simulink model "Project3_System_partB_R2017a"  (R2017a)
settings: Solver=VariableStepAuto  StartTime=0.0  StopTime=10  FixedStep=.001  MaxStep=.001  RelTol=1e-6  EnableMultiTasking=on
values from neighbouring files (symbols this model uses):
  Kd = 700    [SimRun.m]
  Kp = 1000    [SimRun.m]
  n = link.inertia*(iwdot) + cross(iw, link.inertia*iw)    [newtonEuler.m]
  points = points3D    [SimRun.m]
  th_last = [0;-pi/2;0;0;0;0]    [SimRun.m]    (also in fcn.m)
  transPercent = 0.025    [SimRun.m]
(part 4 of 4)

== matlab function Project3_System_partB_R2017a/MATLAB Function ==
  data: theta input; theta_ddot input; torque output; theta_dot input
function torque = newton_euler( theta, theta_ddot, theta_dot )
%#codegen
coder.extrinsic('evalin');
coder.extrinsic('newtonEuler');

persistent linkList boundry_conditions;

if isempty(linkList)
    linkList = evalin('base','linkList');
    boundry_conditions.base_angular_velocity = [0;0;0];
    boundry_conditions.base_angular_acceleration = [0;0;0];
    boundry_conditions.base_linear_acceleration = [0;0;9.8];
    boundry_conditions.distal_force = [0;0;0];
    boundry_conditions.distal_torque = [0;0;0];
end

% theta(2) = theta(2)-pi/2; % put in DH frame
torque = zeros(6,1);
torque = newtonEuler(linkList,theta,theta_dot,theta_ddot,boundry_conditions);


end

== matlab function Project3_System_partB_R2017a/ABB Arm Dynamics/Laser Tracking ==
  data: theta input; pose output
function pose = laserTracker(theta)
%#codegen
coder.extrinsic('evalin');
persistent Sim_Exact;

if isempty(Sim_Exact)
    Sim_Exact = evalin('base','Sim_Exact');
end


th1 = theta(1);
th2 = theta(2);
th3 = theta(3);
th4 = theta(4);
th5 = theta(5);
th6 = theta(6);


if(Sim_Exact)
    pose = [ sin(th6)*(cos(th4)*sin(th1) + sin(th4)*(cos(th1)*sin(th2)*sin(th3) - cos(th1)*cos(th2)*cos(th3))) + cos(th6)*(cos(th5)*(sin(th1)*sin(th4) - cos(th4)*(cos(th1)*sin(th2)*sin(th3) - cos(th1)*cos(th2)*cos(th3))) - sin(th5)*(cos(th1)*cos(th2)*sin(th3) + cos(th1)*cos(th3)*sin(th2))), cos(th6)*(cos(th4)*sin(th1) + sin(th4)*(cos(th1)*sin(th2)*sin(th3) - cos(th1)*cos(th2)*cos(th3))) - sin(th6)*(cos(th5)*(sin(th1)*sin(th4) - cos(th4)*(cos(th1)*sin(th2)*sin(th3) - cos(th1)*cos(th2)*cos(th3))) - sin(th5)*(cos(th1)*cos(th2)*sin(th3) + cos(th1)*cos(th3)*sin(th2))), - sin(th5)*(sin(th1)*sin(th4) - cos(th4)*(cos(th1)*sin(th2)*sin(th3) - cos(th1)*cos(th2)*cos(th3))) - cos(th5)*(cos(th1)*cos(th2)*sin(th3) + cos(th1)*cos(th3)*sin(th2)), (27*cos(th1)*cos(th2))/100 - (9*sin(th5)*(sin(th1)*sin(th4) - cos(th4)*(cos(th1)*sin(th2)*sin(th3) - cos(th1)*cos(th2)*cos(th3))))/125 - (9*cos(th5)*(cos(th1)*cos(th2)*sin(th3) + cos(th1)*cos(th3)*sin(th2)))/125 - (7*cos(th1)*sin(th2)*sin(th3))/100 + (7*cos(th1)*cos(th2)*cos(th3))/100 - (151*cos(th1)*cos(th2)*sin(th3))/500 - (151*cos(th1)*cos(th3)*sin(th2))/500;
        - sin(th6)*(cos(th1)*cos(th4) - sin(th4)*(sin(th1)*sin(th2)*sin(th3) - cos(th2)*cos(th3)*sin(th1))) - cos(th6)*(cos(th5)*(cos(th1)*sin(th4) + cos(th4)*(sin(th1)*sin(th2)*sin(th3) - cos(th2)*cos(th3)*sin(th1))) + sin(th5)*(cos(th2)*sin(th1)*sin(th3) + cos(th3)*sin(th1)*sin(th2))), sin(th6)*(cos(th5)*(cos(th1)*sin(th4) + cos(th4)*(sin(th1)*sin(th2)*sin(th3) - cos(th2)*cos(th3)*sin(th1))) + sin(th5)*(cos(th2)*sin(th1)*sin(th3) + cos(th3)*sin(th1)*sin(th2))) - cos(th6)*(cos(th1)*cos(th4) - sin(th4)*(sin(th1)*sin(th2)*sin(th3) - cos(th2)*cos(th3)*sin(th1))), sin(th5)*(cos(th1)*sin(th4) + cos(th4)*(sin(th1)*sin(th2)*sin(th3) - cos(th2)*cos(th3)*sin(th1))) - cos(th5)*(cos(th2)*sin(th1)*sin(th3) + cos(th3)*sin(th1)*sin(th2)), (27*cos(th2)*sin(th1))/100 + (9*sin(th5)*(cos(th1)*sin(th4) + cos(th4)*(sin(th1)*sin(th2)*sin(th3) - cos(th2)*cos(th3)*sin(th1))))/125 - (9*cos(th5)*(cos(th2)*sin(th1)*sin(th3) + cos(th3)*sin(th1)*sin(th2)))/125 - (151*cos(th2)*sin(th1)*sin(th3))/500 - (151*cos(th3)*sin(th1)*sin(th2))/500 - (7*sin(th1)*sin(th2)*sin(th3))/100 + (7*cos(th2)*cos(th3)*sin(th1))/100;
        sin(th4)*sin(th6)*(cos(th2)*sin(th3) + cos(th3)*sin(th2)) - cos(th6)*(sin(th5)*(cos(th2)*cos(th3) - sin(th2)*sin(th3)) + cos(th4)*cos(th5)*(cos(th2)*sin(th3) + cos(th3)*sin(th2))), sin(th6)*(sin(th5)*(cos(th2)*cos(th3) - sin(th2)*sin(th3)) + cos(th4)*cos(th5)*(cos(th2)*sin(th3) + cos(th3)*sin(th2))) + cos(th6)*sin(th4)*(cos(th2)*sin(th3) + cos(th3)*sin(th2)), cos(th4)*sin(th5)*(cos(th2)*sin(th3) + cos(th3)*sin(th2)) - cos(th5)*(cos(th2)*cos(th3) - sin(th2)*sin(th3)), (151*sin(th2)*sin(th3))/500 - (151*cos(th2)*cos(th3))/500 - (7*cos(th2)*sin(th3))/100 - (7*cos(th3)*sin(th2))/100 - (27*sin(th2))/100 - (9*cos(th5)*(cos(th2)*cos(th3) - sin(th2)*sin(th3)))/125 + (9*cos(th4)*sin(th5)*(cos(th2)*sin(th3) + cos(th3)*sin(th2)))/125 + 29/100;
        0, 0, 0, 1];
else
    
    pose = [ sin(th6)*(cos(th4)*sin(th1) + sin(th4)*(cos(th1)*sin(th2)*sin(th3) - cos(th1)*cos(th2)*cos(th3))) + cos(th6)*(cos(th5)*(sin(th1)*sin(th4) - cos(th4)*(cos(th1)*sin(th2)*sin(th3) - cos(th1)*cos(th2)*cos(th3))) - sin(th5)*(cos(th1)*cos(th2)*sin(th3) + cos(th1)*cos(th3)*sin(th2))), cos(th6)*(cos(th4)*sin(th1) + sin(th4)*(cos(th1)*sin(th2)*sin(th3) - cos(th1)*cos(th2)*cos(th3))) - sin(th6)*(cos(th5)*(sin(th1)*sin(th4) - cos(th4)*(cos(th1)*sin(th2)*sin(th3) - cos(th1)*cos(th2)*cos(th3))) - sin(th5)*(cos(th1)*cos(th2)*sin(th3) + cos(th1)*cos(th3)*sin(th2))), - sin(th5)*(sin(th1)*sin(th4) - cos(th4)*(cos(th1)*sin(th2)*sin(th3) - cos(th1)*cos(th2)*cos(th3))) - cos(th5)*(cos(th1)*cos(th2)*sin(th3) + cos(th1)*cos(th3)*sin(th2)), (151838081588107*cos(th1)*cos(th2))/562949953421312 - (123928564092639*sin(th1))/72057594037927936 - (7184037743251309*cos(th1))/36893488147419103232 - (7330531551818703*cos(th4)*sin(th1))/36893488147419103232 - (5489399374888815*sin(th1)*sin(th4))/9223372036854775808 + (970893499285375*cos(th5)*(sin(th1)*sin(th4) - cos(th4)*(cos(th1)*sin(th2)*sin(th3) - cos(th1)*cos(th2)*cos(th3))))/9223372036854775808 - (5192391675427195*sin(th5)*(sin(th1)*sin(th4) - cos(th4)*(cos(th1)*sin(th2)*sin(th3) - cos(th1)*cos(th2)*cos(th3))))/72057594037927936 + (1663072680156839*sin(th6)*(cos(th4)*sin(th1) + sin(th4)*(cos(th1)*sin(th2)*sin(th3) - cos(th1)*cos(th2)*cos(th3))))/2305843009213693952 + (1663072680156839*cos(th6)*(cos(th5)*(sin(th1)*sin(th4) - cos(th4)*(cos(th1)*sin(th2)*sin(th3) - cos(th1)*cos(th2)*cos(th3))) - sin(th5)*(cos(th1)*cos(th2)*sin(th3) + cos(th1)*cos(th3)*sin(th2))))/2305843009213693952 + (5489399374888815*cos(th4)*(cos(th1)*sin(th2)*sin(th3) - cos(th1)*cos(th2)*cos(th3)))/9223372036854775808 - (5192391675427195*cos(th5)*(cos(th1)*cos(th2)*sin(th3) + cos(th1)*cos(th3)*sin(th2)))/72057594037927936 - (7330531551818703*sin(th4)*(cos(th1)*sin(th2)*sin(th3) - cos(th1)*cos(th2)*cos(th3)))/36893488147419103232 - (970893499285375*sin(th5)*(cos(th1)*cos(th2)*sin(th3) + cos(th1)*cos(th3)*sin(th2)))/9223372036854775808 - (1259578569946919*cos(th1)*sin(th2)*sin(th3))/18014398509481984 + (1259578569946919*cos(th1)*cos(th2)*cos(th3))/18014398509481984 - (5430591396830085*cos(th1)*cos(th2)*sin(th3))/18014398509481984 - (5430591396830085*cos(th1)*cos(th3)*sin(th2))/18014398509481984;
        - sin(th6)*(cos(th1)*cos(th4) - sin(th4)*(sin(th1)*sin(th2)*sin(th3) - cos(th2)*cos(th3)*sin(th1))) - cos(th6)*(cos(th5)*(cos(th1)*sin(th4) + cos(th4)*(sin(th1)*sin(th2)*sin(th3) - cos(th2)*cos(th3)*sin(th1))) + sin(th5)*(cos(th2)*sin(th1)*sin(th3) + cos(th3)*sin(th1)*sin(th2))), sin(th6)*(cos(th5)*(cos(th1)*sin(th4) + cos(th4)*(sin(th1)*sin(th2)*sin(th3) - cos(th2)*cos(th3)*sin(th1))) + sin(th5)*(cos(th2)*sin(th1)*sin(th3) + cos(th3)*sin(th1)*sin(th2))) - cos(th6)*(cos(th1)*cos(th4) - sin(th4)*(sin(th1)*sin(th2)*sin(th3) - cos(th2)*cos(th3)*sin(th1))), sin(th5)*(cos(th1)*sin(th4) + cos(th4)*(sin(th1)*sin(th2)*sin(th3) - cos(th2)*cos(th3)*sin(th1))) - cos(th5)*(cos(th2)*sin(th1)*sin(th3) + cos(th3)*sin(th1)*sin(th2)), (123928564092639*cos(th1))/72057594037927936 - (7184037743251309*sin(th1))/36893488147419103232 + (7330531551818703*cos(th1)*cos(th4))/36893488147419103232 + (151838081588107*cos(th2)*sin(th1))/562949953421312 + (5489399374888815*cos(th1)*sin(th4))/9223372036854775808 - (970893499285375*cos(th5)*(cos(th1)*sin(th4) + cos(th4)*(sin(th1)*sin(th2)*sin(th3) - cos(th2)*cos(th3)*sin(th1))))/9223372036854775808 + (5192391675427195*sin(th5)*(cos(th1)*sin(th4) + cos(th4)*(sin(th1)*sin(th2)*sin(th3) - cos(th2)*cos(th3)*sin(th1))))/72057594037927936 - (1663072680156839*sin(th6)*(cos(th1)*cos(th4) - sin(th4)*(sin(th1)*sin(th2)*sin(th3) - cos(th2)*cos(th3)*sin(th1))))/2305843009213693952 + (5489399374888815*cos(th4)*(sin(th1)*sin(th2)*sin(th3) - cos(th2)*cos(th3)*sin(th1)))/9223372036854775808 - (5192391675427195*cos(th5)*(cos(th2)*sin(th1)*sin(th3) + cos(th3)*sin(th1)*sin(th2)))/72057594037927936 - (1663072680156839*cos(th6)*(cos(th5)*(cos(th1)*sin(th4) + cos(th4)*(sin(th1)*sin(th2)*sin(th3) - cos(th2)*cos(th3)*sin(th1))) + sin(th5)*(cos(th2)*sin(th1)*sin(th3) + cos(th3)*sin(th1)*sin(th2))))/2305843009213693952 - (7330531551818703*sin(th4)*(sin(th1)*sin(th2)*sin(th3) - cos(th2)*cos(th3)*sin(th1)))/36893488147419103232 - (970893499285375*sin(th5)*(cos(th2)*sin(th1)*sin(th3) + cos(th3)*sin(th1)*sin(th2)))/9223372036854775808 - (5430591396830085*cos(th2)*sin(th1)*sin(th3))/18014398509481984 - (5430591396830085*cos(th3)*sin(th1)*sin(th2))/18014398509481984 - (1259578569946919*sin(th1)*sin(th2)*sin(th3))/18014398509481984 + (1259578569946919*cos(th2)*cos(th3)*sin(th1))/18014398509481984;
        sin(th4)*sin(th6)*(cos(th2)*sin(th3) + cos(th3)*sin(th2)) - cos(th6)*(sin(th5)*(cos(th2)*cos(th3) - sin(th2)*sin(th3)) + cos(th4)*cos(th5)*(cos(th2)*sin(th3) + cos(th3)*sin(th2))), sin(th6)*(sin(th5)*(cos(th2)*cos(th3) - sin(th2)*sin(th3)) + cos(th4)*cos(th5)*(cos(th2)*sin(th3) + cos(th3)*sin(th2))) + cos(th6)*sin(th4)*(cos(th2)*sin(th3) + cos(th3)*sin(th2)), cos(th4)*sin(th5)*(cos(th2)*sin(th3) + cos(th3)*sin(th2)) - cos(th5)*(cos(th2)*cos(th3) - sin(th2)*sin(th3)), (5430591396830085*sin(th2)*sin(th3))/18014398509481984 - (5430591396830085*cos(th2)*cos(th3))/18014398509481984 - (1259578569946919*cos(th2)*sin(th3))/18014398509481984 - (1259578569946919*cos(th3)*sin(th2))/18014398509481984 - (1663072680156839*cos(th6)*(sin(th5)*(cos(th2)*cos(th3) - sin(th2)*sin(th3)) + cos(th4)*cos(th5)*(cos(th2)*sin(th3) + cos(th3)*sin(th2))))/2305843009213693952 - (151838081588107*sin(th2))/562949953421312 + (5489399374888815*cos(th4)*(cos(th2)*sin(th3) + cos(th3)*sin(th2)))/9223372036854775808 - (5192391675427195*cos(th5)*(cos(th2)*cos(th3) - sin(th2)*sin(th3)))/72057594037927936 - (7330531551818703*sin(th4)*(cos(th2)*sin(th3) + cos(th3)*sin(th2)))/36893488147419103232 - (970893499285375*sin(th5)*(cos(th2)*cos(th3) - sin(th2)*sin(th3)))/9223372036854775808 - (970893499285375*cos(th4)*cos(th5)*(cos(th2)*sin(th3) + cos(th3)*sin(th2)))/9223372036854775808 + (5192391675427195*cos(th4)*sin(th5)*(cos(th2)*sin(th3) + cos(th3)*sin(th2)))/72057594037927936 + (1663072680156839*sin(th4)*sin(th6)*(cos(th2)*sin(th3) + cos(th3)*sin(th2)))/2305843009213693952 + 325695105792877/1125899906842624;
        0, 0, 0, 1];
end

== matlab function Project3_System_partB_R2017a/MATLAB Function1 ==
  data: t input; traj output; points input; n input
function traj = trajectory(t,points,n)
d1 = 0.29;
a2 = 0.270;
a3 = 0.070;
d4 = 0.302;
d6 = 0.072;

rcom1 = [0;-d1/2;0];
rcom2 = [-a2/2;0;0];
rcom3 = [-a3/2;0;0];
rcom4 = [0;-d4/2;0];
rcom5 = [0;0;0];
rcom6 = [0; -d6/2;0];

rad1 = .2/2; h1 = d1;   m1 = 8050*h1*rad1^2*pi;
rad2 = .15/2; h2 = a2;   m2 = 8050*h2*rad2^2*pi;
rad3 = .1/2; h3 = a3;  m3 = 8050*h3*rad3^2*pi;
rad4 = .1/2; h4 = d4;  m4 = 8050*h4*rad4^2*pi;
rad5 = .05/2; h5 = .125; m5 = 8050*h5*rad5^2*pi;
rad6 = .05/2; h6 = d6;  m6 = 8050*h6*rad6^2*pi;

J1 = diag(m1*[1/12*(3*rad1^2+h1^2),rad1^2/2,1/12*(3*rad1^2+h1^2)]);
J2 = diag(m2*[rad2^2/2,1/12*(3*rad2^2+h2^2),1/12*(3*rad2^2+h2^2)]);
J3 = diag(m3*[rad3^2/2,1/12*(3*rad3^2+h3^2),1/12*(3*rad3^2+h3^2)]);
J4 = diag(m4*[1/12*(3*rad4^2+h4^2),rad4^2/2,1/12*(3*rad4^2+h4^2)]);
J5 = diag(m5*[1/12*(3*rad5^2+h5^2),rad5^2/2,1/12*(3*rad5^2+h5^2)]);
J6 = diag(m6*[1/12*(3*rad6^2+h6^2),rad6^2/2,1/12*(3*rad6^2+h6^2)]);

L1 = createLink(0,d1,-pi/2,[],rcom1, m1,J1);
L2 = createLink(a2,0,0,[],rcom2, m2,J2);
L3 = createLink(a3,0,-pi/2,[],rcom3, m3,J3);
L4 = createLink(0,d4,pi/2,[],rcom4, m4,J4);
L5 = createLink(0,0,-pi/2,[],rcom5, m5,J5);
L6 = createLink(0,d6,0,[],rcom6, m6,J6);

linkList = [L1;L2;L3;L4;L5;L6]';

traj=zeros(length(t),8);
traj1=zeros(length(t),8);
% [p,~]=size(points);
% th=zeros(p+3,6);
% th(1,:)=[0;pi/2;0;0;0;0]';
z_vec=n;
Q=zeros(4,length(t));
Q1=zeros(4,length(t));
% H_ini=dhFwdKine(linkList,th(1,:));
% R_ini=H_ini(1:3,1:3);
Q1(:,1) = rot2Quat(eye(3));
Q(:,1)=Q1(:,1)/norm(Q1(:,1));
diff=(points(2,:)-points(1,:));
x_vec=diff'/norm(diff);
y_vec=cpMap(z_vec)*x_vec;
R=[x_vec y_vec z_vec];
traj1(1,:)=[t(1),[0 0 0],Q(:,1)'];
% [th1,th2,th3,th4,th5,th6 ,~]=abbInvKine([eye(3) points(1,:)'],-1*th(1,:)');
% th(2,:)=[th1,th2,th3,th4,th5,th6];
% th(3,:)=[th1,th2,th3,th4,th5,th6];
% H_i=dhFwdKine(linkList,th(2,:)');
% R_i=H_i(1:3,1:3);
Q1(:,2) = rot2Quat(R);
Q(:,2)=Q1(:,2)/norm(Q1(:,2));
traj1(2,:)=[t(2),points(1,:),Q(:,2)'];
traj1(3,:)=[t(3),points(1,:),Q(:,2)'];
for i=3:length(t)-2
    diff=points(i-1,:)-points(i-2,:);
    x_vec=diff'/norm(diff);
    y_vec=cpMap(z_vec)*x_vec;
    R=[x_vec y_vec z_vec];
% [th1,th2,th3,th4,th5,th6 ,~]=abbInvKine([eye(3) points(i-1,:)'],th(i,:)');
% th(i+1,:)=[th1,th2,th3,th4,th5,th6];
% H_i=dhFwdKine(linkList,th(i,:)');
% R_i=H_i(1:3,1:3);
Q1(:,i) = rot2Quat(R);
Q(:,i)=Q1(:,i)/norm(Q1(:,i));
if (Q(:,i-1)')*Q(:,i) < 0
    Q=-1*Q;
end
traj1(i+1,:)=[t(i+1),points(i-1,:),Q(:,i)'];
end
traj1(24,:)=[t(24),points(21,:),Q(:,i)'];
traj=traj1;
end

== matlab function Project3_System_partB_R2017a/MATLAB Function2 ==
  data: time input double; T_des output double; x_des_ddot output; traj input double; transPercent input double; x_des_dot output double
function [T_des,x_des_ddot,x_des_dot] = constAccelInterp(time,traj,transPercent)
t = traj(:,1);
[n,m] = size(traj);
x1 = zeros(1,7);
x1_dot = zeros(1,7);
x1_ddot = zeros(1,7);
omega=zeros(3,1);
omega1=zeros(3,1);
x_des=zeros(6,1);
x_dot_des=zeros(6,1);
q1=zeros(4,1);
q=zeros(4,1);

for j = 2:n-1
    if j-1==1 && time>=t(j-1,1) && time<=(t(j-1,1)+transPercent)
        for i = 2:m
            x1(1,i-1) = traj(j-1,i) + (((traj(j,i)-traj(j-1,i))*((time-t(j-1,1)+transPercent)^2))/(4*transPercent*(t(j,1)-t(j-1,1))));
            x1_dot(1,i-1) = (((traj(j,i)-traj(j-1,i))*(time-t(j-1,1)+transPercent))/(2*transPercent*(t(j,1)-t(j-1,1))));
            x1_ddot(1,i-1) = ((traj(j,i)-traj(j-1,i))/(2*transPercent*(t(j,1)-t(j-1,1))));
        end
        break;
    elseif j+1==n && time>=(t(j+1,1)-transPercent) && time<=t(j+1,1)
        for i = 2:m
            x1(1,i-1) = traj(j+1,i) - (((traj(j+1,i)-traj(j,i))*((time-t(j+1,1)-transPercent)^2))/(4*transPercent*(t(j+1,1)-t(j,1))));
            x1_dot(1,i-1) = -(((traj(j+1,i)-traj(j,i))*(time-t(j+1,1)-transPercent))/(2*transPercent*(t(j+1,1)-t(j,1))));
            x1_ddot(1,i-1) = -((traj(j+1,i)-traj(j,i))/(2*transPercent*(t(j+1,1)-t(j,1))));
        end
        break;
    elseif time>=(t(j-1,1)+transPercent) && time<=(t(j,1)-transPercent)
        for i = 2:m
            x1(1,i-1) = traj(j,i)-(((t(j,1)-time)*(traj(j,i)- traj(j-1,i)))/(t(j,1)-t(j-1,1)));
            x1_dot(1,i-1) = (traj(j,i)-traj(j-1,i))/(t(j,1)-t(j-1,1));
            x1_ddot(1,i-1) = 0.0;
        end
        break;
    elseif time>=(t(j,1)-transPercent) && time<=(t(j,1)+transPercent)
        for i = 2:m
            x1(1,i-1) = traj(j,i) - ...
                (((traj(j,i)-traj(j-1,i))*((time-t(j,1)-transPercent)^2))/(4*transPercent*(t(j,1)-t(j-1,1)))) + (((traj(j+1,i)-traj(j,i))*((time-t(j,1)+transPercent)^2))/(4*transPercent*(t(j+1,1)-t(j,1))));
            x1_dot(1,i-1) = -(((traj(j,i)-traj(j-1,i))*(time-t(j,1)-transPercent))/(2*transPercent*(t(j,1)-t(j-1,1)))) + (((traj(j+1,i)-traj(j,i))*(time-t(j,1)+transPercent))/(2*transPercent*(t(j+1,1)-t(j,1))));
            x1_ddot(1,i-1) = -((traj(j,i)-traj(j-1,i))/(2*transPercent*(t(j,1)-t(j-1,1)))) + ((traj(j+1,i)-traj(j,i))/(2*transPercent*(t(j+1,1)-t(j,1))));
        end
        break;
    elseif time>=(t(j,1)+transPercent) && time<=(t(j+1,1)-transPercent)
        for i = 2:m
            x1(1,i-1) = traj(j,i)+(((time-t(j,1))*(traj(j+1,i)-traj(j,i)))/(t(j+1,1)-t(j,1)));
            x1_dot(1,i-1) = (traj(j+1,i)-traj(j,i))/(t(j+1,1)-t(j,1));
            x1_ddot(1,i-1) = 0;
        end
        break;
        
    end
end
q1(:,1)=x1(4:7)';
R=quat2Rot(q1);
% [k,theta]=rot2AngleAxis(R);
% omega=k*theta;
T_des=[R x1(1:3)';0 0 0 1];
% x_des=[x1(1:3),omega']';
dq=x1_dot(4:7);
omega1=2*[dq(2:4)' (dq(1)*eye(3))+cpMap(dq(2:4))]*dq';
x_des_dot=[x1_dot(1:3)';omega1]';
dq1=x1_ddot(4:7);
omega_dot=2*[dq1(2:4)' (dq1(1)*eye(3))+cpMap(dq1(2:4))]*dq1';
x_des_ddot=[x1_ddot(1:3)';omega_dot]';
end

== matlab function Project3_System_partB_R2017a/MATLAB Function3 ==
  data: Jv output; paramList input; paramRateList input; Jv_inv output; JvDot output
function [Jv,Jv_inv,JvDot] = Jacobian(paramList,paramRateList)

d1 = 0.29;
a2 = 0.270;
a3 = 0.070;
d4 = 0.302;
d6 = 0.072;

rcom1 = [0;-d1/2;0];
rcom2 = [-a2/2;0;0];
rcom3 = [-a3/2;0;0];
rcom4 = [0;-d4/2;0];
rcom5 = [0;0;0];
rcom6 = [0; -d6/2;0];

rad1 = .2/2; h1 = d1;   m1 = 8050*h1*rad1^2*pi;
rad2 = .15/2; h2 = a2;   m2 = 8050*h2*rad2^2*pi;
rad3 = .1/2; h3 = a3;  m3 = 8050*h3*rad3^2*pi;
rad4 = .1/2; h4 = d4;  m4 = 8050*h4*rad4^2*pi;
rad5 = .05/2; h5 = .125; m5 = 8050*h5*rad5^2*pi;
rad6 = .05/2; h6 = d6;  m6 = 8050*h6*rad6^2*pi;

J1 = diag(m1*[1/12*(3*rad1^2+h1^2),rad1^2/2,1/12*(3*rad1^2+h1^2)]);
J2 = diag(m2*[rad2^2/2,1/12*(3*rad2^2+h2^2),1/12*(3*rad2^2+h2^2)]);
J3 = diag(m3*[rad3^2/2,1/12*(3*rad3^2+h3^2),1/12*(3*rad3^2+h3^2)]);
J4 = diag(m4*[1/12*(3*rad4^2+h4^2),rad4^2/2,1/12*(3*rad4^2+h4^2)]);
J5 = diag(m5*[1/12*(3*rad5^2+h5^2),rad5^2/2,1/12*(3*rad5^2+h5^2)]);
J6 = diag(m6*[1/12*(3*rad6^2+h6^2),rad6^2/2,1/12*(3*rad6^2+h6^2)]);

L1 = createLink(0,d1,-pi/2,[],rcom1, m1,J1);
L2 = createLink(a2,0,0,[],rcom2, m2,J2);
L3 = createLink(a3,0,-pi/2,[],rcom3, m3,J3);
L4 = createLink(0,d4,pi/2,[],rcom4, m4,J4);
L5 = createLink(0,0,-pi/2,[],rcom5, m5,J5);
L6 = createLink(0,d6,0,[],rcom6, m6,J6);

linkList = [L1;L2;L3;L4;L5;L6]';

Jv=zeros(6,6);
JvDot=zeros(6,6);
Jv_inv=zeros(6,6);
[Jv, JvDot]= velocityJacobian(linkList, paramList, paramRateList);
[U,S,V] = svd(Jv);
    Sinv = S';
    Sinv(Sinv/Sinv(1,1) > sqrt(eps)) = 1./Sinv(Sinv/Sinv(1,1) > sqrt(eps));
    Sinv(1./Sinv < sqrt(eps)) = 0;
    Jv_inv = (V)*Sinv*(U');

== matlab function Project3_System_partB_R2017a/MATLAB Function4 ==
  data: Jv_inv input; u input; gain output
 function gain = Jv_inv(Jv_inv,u)
gain=zeros(1,6);
gain1 = Jv_inv*u';
gain=gain1';
end

== matlab function Project3_System_partB_R2017a/MATLAB Function5 ==
  data: JvDot input; u input; gain output
function gain = JvDot(JvDot,u)
gain=zeros(1,6);
gain1 = JvDot*u;
gain=gain1';
end

== matlab function Project3_System_partB_R2017a/MATLAB Function6 ==
  data: Jv input; u input; gain output
function gain = Jv(Jv,u)
gain=zeros(1,6);
gain1 = Jv*u;
gain=gain1';
end

== matlab function Project3_System_partB_R2017a/MATLAB Function7 ==
  data: theta input; Y output
function Y = fwdKine(theta)
d1 = 0.29;
a2 = 0.270;
a3 = 0.070;
d4 = 0.302;
d6 = 0.072;

rcom1 = [0;-d1/2;0];
rcom2 = [-a2/2;0;0];
rcom3 = [-a3/2;0;0];
rcom4 = [0;-d4/2;0];
rcom5 = [0;0;0];
rcom6 = [0; -d6/2;0];

rad1 = .2/2; h1 = d1;   m1 = 8050*h1*rad1^2*pi;
rad2 = .15/2; h2 = a2;   m2 = 8050*h2*rad2^2*pi;
rad3 = .1/2; h3 = a3;  m3 = 8050*h3*rad3^2*pi;
rad4 = .1/2; h4 = d4;  m4 = 8050*h4*rad4^2*pi;
rad5 = .05/2; h5 = .125; m5 = 8050*h5*rad5^2*pi;
rad6 = .05/2; h6 = d6;  m6 = 8050*h6*rad6^2*pi;

J1 = diag(m1*[1/12*(3*rad1^2+h1^2),rad1^2/2,1/12*(3*rad1^2+h1^2)]);
J2 = diag(m2*[rad2^2/2,1/12*(3*rad2^2+h2^2),1/12*(3*rad2^2+h2^2)]);
J3 = diag(m3*[rad3^2/2,1/12*(3*rad3^2+h3^2),1/12*(3*rad3^2+h3^2)]);
J4 = diag(m4*[1/12*(3*rad4^2+h4^2),rad4^2/2,1/12*(3*rad4^2+h4^2)]);
J5 = diag(m5*[1/12*(3*rad5^2+h5^2),rad5^2/2,1/12*(3*rad5^2+h5^2)]);
J6 = diag(m6*[1/12*(3*rad6^2+h6^2),rad6^2/2,1/12*(3*rad6^2+h6^2)]);

L1 = createLink(0,d1,-pi/2,[],rcom1, m1,J1);
L2 = createLink(a2,0,0,[],rcom2, m2,J2);
L3 = createLink(a3,0,-pi/2,[],rcom3, m3,J3);
L4 = createLink(0,d4,pi/2,[],rcom4, m4,J4);
L5 = createLink(0,0,-pi/2,[],rcom5, m5,J5);
L6 = createLink(0,d6,0,[],rcom6, m6,J6);

linkList = [L1;L2;L3;L4;L5;L6]';

X1=zeros(3,1);
k=zeros(3,1);
omega=zeros(3,1);
Y=zeros(4,4);

Y=dhFwdKine(linkList,theta);
% R=Y(1:3,1:3);
% [k, theta1] = rot2AngleAxis(R);
% omega=theta1*k;
% X1=Y(1:3,4);
% X=[X1;omega];
end

== matlab function Project3_System_partB_R2017a/MATLAB Function8 ==
  data: Tc input; Td input; error_vector output
function error_vector  = transError(Tc,Td)
d_Des = Td(1:3,4);
d_Cur = Tc(1:3,4);
position_error = d_Des - d_Cur;
rot_error = rotationError(Td(1:3,1:3),Tc(1:3,1:3));
error_vector = [position_error;rot_error];
end
